simulink model "Lecture4Exercise"  (R2020b)
settings: Solver=VariableStepAuto  StartTime=0.0  StopTime=10  RelTol=1e-3
values from neighbouring files (symbols this model uses):
  Ad = [0.8, -0.36; 0.09, 0.98]    [Lecture4Exercise.m]
  Bd = [0.09; 0.0047]    [Lecture4Exercise.m]
  Cd = [0, 10]    [Lecture4Exercise.m]    (also in Lecture5Exercises.m = C; Lecture6Exercise.m = C)
  Dd = [0; 0]    [Lecture4Exercise.m]    (also in Lecture5Exercises.m = 0; Lecture6Exercise.m = 0)
  K = [KKi(1) KKi(2)]    [Lecture4Exercise.m]    (also in Lecture5Exercises.m = acker(A_adj, B_adj, [z_p z_p z_p]); Lecture9Exercise.m = P\D)
  Ki = 27    [Lecture10_11Exercise.m]    (also in Lecture4Exercise.m = -KKi(3))
  Lc = acker(Ad', (Cd*Ad)', [z_pe, z_pe])'    [Lecture4Exercise.m]
  T = 0.1    [Lecture10_11Exercise.m]    (also in Lecture4Exercise.m)
settings Model: Creator=sebastian  LastModifiedBy=sebastian

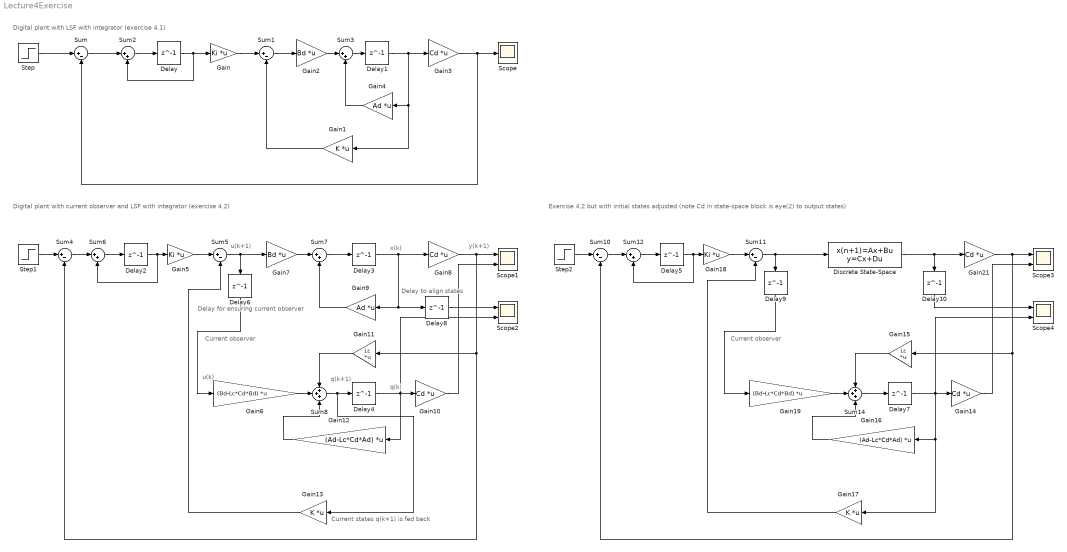
== system Lecture4Exercise ==
  note: Current states q(k+1) is fed back
  note: x(k)
  note: q(k+1)
  note: u(k+1)
  note: u(k)
  note: q(k)
  note: y(k+1)
  note: Delay to align states
  note: Delay for ensuring current observer
  note: Digital plant with LSF with integrator (exercise 4.1)
  note: Digital plant with current observer and LSF with integrator (exercise 4.2)
  note: Current observer
  note: Current observer
  note: Exercise 4.2 but with initial states adjusted (note Cd in state-space block is eye(2) to output states)
  Delay{,1..5,7} (7 alike) : Delay  DelayLength=1  InitialCondition=0  SampleTime=T
  Delay{6,8..10} (4 alike) : Delay  DelayLength=1  SampleTime=T
  Discrete State-Space : DiscreteStateSpace  A=Ad  B=Bd  C=eye(2)  D=Dd  SampleTime=T
  Gain : Gain  Gain=Ki  Multiplication=Matrix(K*u)
  Gain1 : Gain  Gain=K  Multiplication=Matrix(K*u)
  Gain{3,8,10,14,21} (5 alike) : Gain  Gain=Cd  Multiplication=Matrix(K*u)
  Gain11 : Gain  Gain=Lc  Multiplication=Matrix(K*u)
  Gain12 : Gain  Gain=(Ad-Lc*Cd*Ad)  Multiplication=Matrix(K*u)
  Gain13 : Gain  Gain=K  Multiplication=Matrix(K*u)
  Gain15 : Gain  Gain=Lc  Multiplication=Matrix(K*u)
  Gain16 : Gain  Gain=(Ad-Lc*Cd*Ad)  Multiplication=Matrix(K*u)
  Gain17 : Gain  Gain=K  Multiplication=Matrix(K*u)
  Gain18 : Gain  Gain=Ki  Multiplication=Matrix(K*u)
  Gain19 : Gain  Gain=(Bd-Lc*Cd*Bd)  Multiplication=Matrix(K*u)
  Gain2 : Gain  Gain=Bd  Multiplication=Matrix(K*u)
  Gain4 : Gain  Gain=Ad  Multiplication=Matrix(K*u)
  Gain5 : Gain  Gain=Ki  Multiplication=Matrix(K*u)
  Gain6 : Gain  Gain=(Bd-Lc*Cd*Bd)  Multiplication=Matrix(K*u)
  Gain7 : Gain  Gain=Bd  Multiplication=Matrix(K*u)
  Gain9 : Gain  Gain=Ad  Multiplication=Matrix(K*u)
  Scope : Scope
  Scope{1..4} (4 alike) : Scope  NumInputPorts=2
  Step : Step  Time=0  SampleTime=0
  Step1 : Step  Time=0  SampleTime=0
  Step2 : Step  Time=0  SampleTime=0
  Sum{,1,4..5,10..11} (6 alike) : Sum  Inputs=|+-
  Sum{2..3,6..7,12} (5 alike) : Sum  Inputs=|++
  Sum14 : Sum  Inputs=+++
  Sum8 : Sum  Inputs=+++
  wires:
  Step/1 -> Sum/1
  Gain/1 -> Sum1/1
  Sum/1 -> Sum2/1
  Sum2/1 -> Delay/1
  Delay/1 -> Sum2/2, Gain/1
  Gain1/1 -> Sum1/2
  Sum1/1 -> Gain2/1
  Gain2/1 -> Sum3/1
  Sum3/1 -> Delay1/1
  Gain4/1 -> Sum3/2
  Delay1/1 -> Gain4/1, Gain1/1, Gain3/1
  Gain3/1 -> Sum/2, Scope/1
  Delay2/1 -> Sum6/2, Gain5/1
  Sum7/1 -> Delay3/1
  Gain5/1 -> Sum5/1
  Gain7/1 -> Sum7/1
  Step1/1 -> Sum4/1
  Sum5/1 -> Gain7/1, Delay6/1
  Gain9/1 -> Sum7/2
  Sum6/1 -> Delay2/1
  Sum4/1 -> Sum6/1
  Gain6/1 -> Sum8/2
  Sum8/1 -> Gain13/1, Delay4/1
  Gain8/1 -> Gain11/1, Sum4/2, Scope1/1
  Gain11/1 -> Sum8/1
  Gain12/1 -> Sum8/3
  Gain13/1 -> Sum5/2
  Delay4/1 -> Gain12/1, Scope2/2, Gain10/1
  Sum12/1 -> Delay5/1
  Sum10/1 -> Sum12/1
  Step2/1 -> Sum10/1
  Gain18/1 -> Sum11/1
  Sum14/1 -> Delay7/1
  Sum11/1 -> Discrete State-Space/1, Delay9/1
  Gain17/1 -> Sum11/2
  Delay7/1 -> Gain16/1, Gain17/1, Scope4/2, Gain14/1
  Gain19/1 -> Sum14/2
  Delay5/1 -> Sum12/2, Gain18/1
  Gain21/1 -> Gain15/1, Sum10/2, Scope3/1
  Gain16/1 -> Sum14/3
  Gain15/1 -> Sum14/1
  Discrete State-Space/1 -> Delay10/1, Gain21/1
  Delay6/1 -> Gain6/1
  Gain10/1 -> Scope1/2
  Delay3/1 -> Gain9/1, Delay8/1, Gain8/1
  Gain14/1 -> Scope3/2
  Delay9/1 -> Gain19/1
  Delay10/1 -> Scope4/1
  Delay8/1 -> Scope2/1
